simulink model "ShipWareDynamics"  (R2020b)
settings: Solver=ode5  StartTime=0.0  StopTime=120  FixedStep=0.001  RelTol=1e-3
undefined symbols (not defined in the file): a, dphi0, K, phi0, T, u0, x0, y0
settings Model: Creator=Hu  LastModifiedBy=chuanhui
settings SFSimCC: CustomCodeUndefinedFunction=UseInterfaceOnly

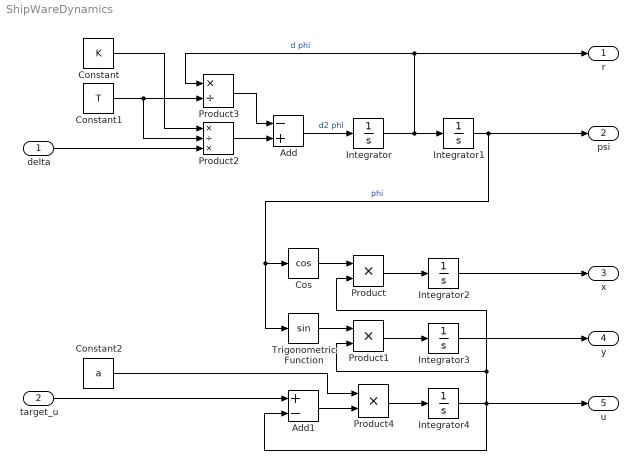
== system ShipWareDynamics ==
  delta : Inport
  target_u : Inport  Port=2
  Add : Sum  Inputs=-+
  Add1 : Sum  Inputs=+-
  Constant : Constant  Value=K
  Constant1 : Constant  Value=T
  Constant2 : Constant  Value=a
  Cos : Trigonometry  Operator=cos
  Integrator : Integrator  InitialCondition=dphi0
  Integrator1 : Integrator  InitialCondition=phi0
  Integrator2 : Integrator  InitialCondition=x0
  Integrator3 : Integrator  InitialCondition=y0
  Integrator4 : Integrator  InitialCondition=u0
  Product : Product
  Product1 : Product
  Product2 : Product  Inputs=*/*
  Product3 : Product  Inputs=*/
  Product4 : Product  Inputs=**
  Trigonometric Function : Trigonometry
  r : Outport  Unit=rad/s  VectorParamsAs1DForOutWhenUnconnected=off
  psi : Outport  Port=2  Unit=rad  VectorParamsAs1DForOutWhenUnconnected=off
  x : Outport  Port=3  Unit=m  VectorParamsAs1DForOutWhenUnconnected=off
  y : Outport  Port=4  Unit=m  VectorParamsAs1DForOutWhenUnconnected=off
  u : Outport  Port=5  Unit=m/s  VectorParamsAs1DForOutWhenUnconnected=off
  wires:
  Product2/1 -> Add/2
  Integrator2/1 -> x/1
  Product3/1 -> Add/1
  Product/1 -> Integrator2/1
  Product1/1 -> Integrator3/1
  Integrator1/1 -> psi/1, Trigonometric Function/1, Cos/1  "phi"
  Add1/1 -> Product4/2
  Add/1 -> Integrator/1  "d2 phi"
  Integrator/1 -> Product3/1, r/1, Integrator1/1  "d phi"
  delta/1 -> Product2/3
  Integrator4/1 -> Product1/2, Product/2, Add1/2, u/1
  Trigonometric Function/1 -> Product1/1
  Integrator3/1 -> y/1
  Product4/1 -> Integrator4/1
  target_u/1 -> Add1/1
  Cos/1 -> Product/1
  Constant1/1 -> Product3/2, Product2/2
  Constant/1 -> Product2/1
  Constant2/1 -> Product4/1
